simulink model "test(1)"  (R2019a)
settings: Solver=FixedStepAuto  StartTime=0.0  StopTime=inf  RelTol=1e-3
libraries: vexarmcortexlib x23, vexcommonlib x3
settings Model: Creator=hsstudent  LastModifiedBy=hsstudent
settings SolverCC: AutoInsertRateTranBlk=on
settings DataIOCC: LimitDataPoints=on  SignalLoggingSaveFormat=ModelDataLogs  ReturnWorkspaceOutputs=off
settings OptimizationCC: ExpressionDepthLimit=2147483647  LifeSpan=Inf  MaxStackSize=64
settings DebuggingCC: UnderspecifiedInitializationDetection=Classic  MergeDetectMultiDrivingBlocksExec=none  InheritedTsInSrcMsg=none  FcnCallInpInsideContextMsg=warning  UnconnectedInputMsg=none  UnconnectedOutputMsg=none  StateNameClashWarn=warning  SFUnexpectedBacktrackingDiag=warning  SFNoUnconditionalDefaultTransitionDiag=warning  SFExecutionAtInitializationDiag=none  ArithmeticOperatorsInVariantConditions=warning
settings HardwareCC: ProdBitPerPointer=32  ProdBitPerSizeT=32  ProdBitPerPtrDiffT=32  ProdLargestAtomicInteger=Long  ProdLargestAtomicFloat=Double  ProdIntDivRoundTo=Undefined  ProdWordSize=32  ProdHWDeviceType=ARM Compatible->ARM Cortex
settings ModelReferenceCC: PropagateSignalLabelsOutOfModel=off
settings SFSimCC: MATLABDynamicMemAlloc=off
settings RTWCC: SystemTargetFile=ert.tlc  HardwareBoard=ARM Cortex-based VEX Microcontroller  TemplateMakefile=ert_default_tmf  Toolchain=GNU Tools for VEX ARM Cortex
settings CodeAppCC: IgnoreCustomStorageClasses=off  CustomSymbolStrType=$N$R$M  StateflowObjectComments=on  InternalIdentifier=Classic
settings ERTTargetCC: CodeReplacementLibrary=GCC ARM Cortex-M3  MultiwordLength=2048  ConvertIfToSwitch=off  SuppressUnreachableDefaultCases=off

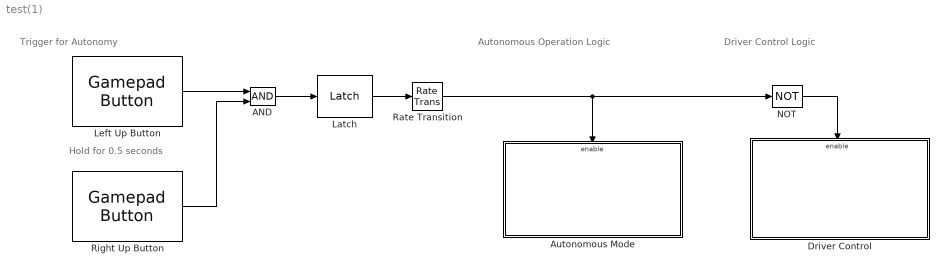
== system test(1) ==
  note: Autonomous Operation Logic
  note: Hold for 0.5 seconds
  note: Driver Control Logic
  note: Trigger for Autonomy
  AND : Logic  IconShape=distinctive  AllPortsSameDT=off  OutDataTypeStr=boolean
  Autonomous Mode : Subsystem
  Driver Control : Subsystem  TreatAsAtomicUnit=on
  Latch : vexcommonlib/Latch  output0=off  BlockPlatform=vexarmcortex
      settings: SourceProductName=Simulink Coder Support Package for ARM Cortex-based VEX Microcontroller  SourceProductBaseCode=EC_VEX_MICRO
  Left Up Button : vexarmcortexlib/Gamepad/Gamepad Button  joystick=1  chan=7  button56=Down  button78=Up  SimulationIn=off  SampleTime=0.5
      settings: SourceProductName=Simulink Coder Support Package for ARM Cortex-based VEX Microcontroller  SourceProductBaseCode=EC_VEX_MICRO
  NOT : Logic  Operator=NOT  IconShape=distinctive  AllPortsSameDT=off  OutDataTypeStr=boolean
  Rate Transition : RateTransition
  Right Up Button : vexarmcortexlib/Gamepad/Gamepad Button  joystick=1  chan=8  button56=Down  button78=Up  SimulationIn=off  SampleTime=0.5
      settings: SourceProductName=Simulink Coder Support Package for ARM Cortex-based VEX Microcontroller  SourceProductBaseCode=EC_VEX_MICRO
  wires:
  AND/1 -> Latch/1
  Rate Transition/1 -> NOT/1, Autonomous Mode/Enable
  Latch/1 -> Rate Transition/1
  Right Up Button/1 -> AND/2
  Left Up Button/1 -> AND/1
  NOT/1 -> Driver Control/Enable

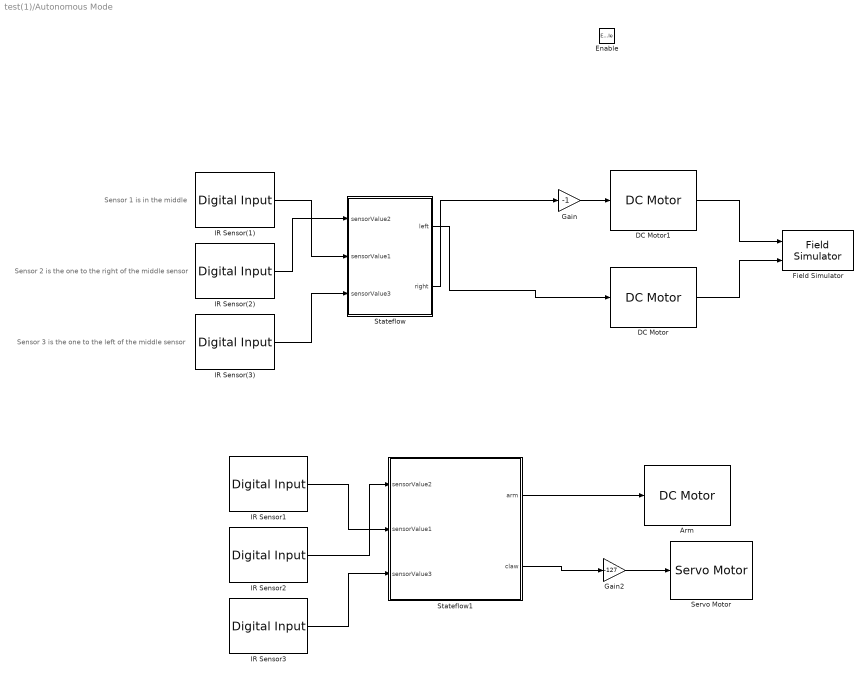
== system test(1)/Autonomous Mode ==
  note: Sensor 3 is the one to the left of the middle sensor
  note: Sensor 2 is the one to the right of the middle sensor
  note: Sensor 1 is in the middle
  Enable : EnablePort  StatesWhenEnabling=reset
  Arm : vexarmcortexlib/Actuators/DC Motor  motor=7  scaleFactor=1/13.5  SimulationOut=on
      settings: SourceProductName=Simulink Coder Support Package for ARM Cortex-based VEX Microcontroller  SourceProductBaseCode=EC_VEX_MICRO
  DC Motor : vexarmcortexlib/Actuators/DC Motor  motor=3  scaleFactor=1/13.5  SimulationOut=on
      settings: SourceProductName=Simulink Coder Support Package for ARM Cortex-based VEX Microcontroller  SourceProductBaseCode=EC_VEX_MICRO
  DC Motor1 : vexarmcortexlib/Actuators/DC Motor  motor=2  scaleFactor=1/13.5  SimulationOut=on
      settings: SourceProductName=Simulink Coder Support Package for ARM Cortex-based VEX Microcontroller  SourceProductBaseCode=EC_VEX_MICRO
  Field Simulator : vexcommonlib/Field Simulator  radius=2.5  space=10  range=200  BlockPlatform=vexarmcortex
      settings: SourceProductName=Simulink Coder Support Package for ARM Cortex-based VEX Microcontroller  SourceProductBaseCode=EC_VEX_MICRO
  Gain : Gain  Gain=-1
  Gain2 : Gain  Gain=-127
  IR Sensor(1) : vexarmcortexlib/Sensors/Digital Input  inChan=9  SimulationIn=off  SampleTime=0.05
      settings: SourceProductName=Simulink Coder Support Package for ARM Cortex-based VEX Microcontroller  SourceProductBaseCode=EC_VEX_MICRO
  IR Sensor(2) : vexarmcortexlib/Sensors/Digital Input  inChan=8  SimulationIn=off  SampleTime=0.05
      settings: SourceProductName=Simulink Coder Support Package for ARM Cortex-based VEX Microcontroller  SourceProductBaseCode=EC_VEX_MICRO
  IR Sensor(3) : vexarmcortexlib/Sensors/Digital Input  inChan=7  SimulationIn=off  SampleTime=0.05
      settings: SourceProductName=Simulink Coder Support Package for ARM Cortex-based VEX Microcontroller  SourceProductBaseCode=EC_VEX_MICRO
  IR Sensor1 : vexarmcortexlib/Sensors/Digital Input  inChan=9  SimulationIn=off  SampleTime=0.05
      settings: SourceProductName=Simulink Coder Support Package for ARM Cortex-based VEX Microcontroller  SourceProductBaseCode=EC_VEX_MICRO
  IR Sensor2 : vexarmcortexlib/Sensors/Digital Input  inChan=8  SimulationIn=off  SampleTime=0.05
      settings: SourceProductName=Simulink Coder Support Package for ARM Cortex-based VEX Microcontroller  SourceProductBaseCode=EC_VEX_MICRO
  IR Sensor3 : vexarmcortexlib/Sensors/Digital Input  inChan=7  SimulationIn=off  SampleTime=0.05
      settings: SourceProductName=Simulink Coder Support Package for ARM Cortex-based VEX Microcontroller  SourceProductBaseCode=EC_VEX_MICRO
  Servo Motor : vexarmcortexlib/Actuators/Servo Motor  motor=4  scaleFactor=60/127  SimulationOut=on
      settings: SourceProductName=Simulink Coder Support Package for ARM Cortex-based VEX Microcontroller  SourceProductBaseCode=EC_VEX_MICRO
  Stateflow : Stateflow chart  TreatAsAtomicUnit=on
  Stateflow1 : Stateflow chart  TreatAsAtomicUnit=on
  wires:
  DC Motor/1 -> Field Simulator/2
  Gain/1 -> DC Motor1/1
  DC Motor1/1 -> Field Simulator/1
  Stateflow/1(left) -> DC Motor/1
  Stateflow/2(right) -> Gain/1
  IR Sensor(1)/1 -> Stateflow/2(sensorValue1)
  IR Sensor1/1 -> Stateflow1/2(sensorValue1)
  IR Sensor2/1 -> Stateflow1/1(sensorValue2)
  IR Sensor3/1 -> Stateflow1/3(sensorValue3)
  Stateflow1/1(arm) -> Arm/1
  Gain2/1 -> Servo Motor/1
  Stateflow1/2(claw) -> Gain2/1
  IR Sensor(2)/1 -> Stateflow/1(sensorValue2)
  IR Sensor(3)/1 -> Stateflow/3(sensorValue3)

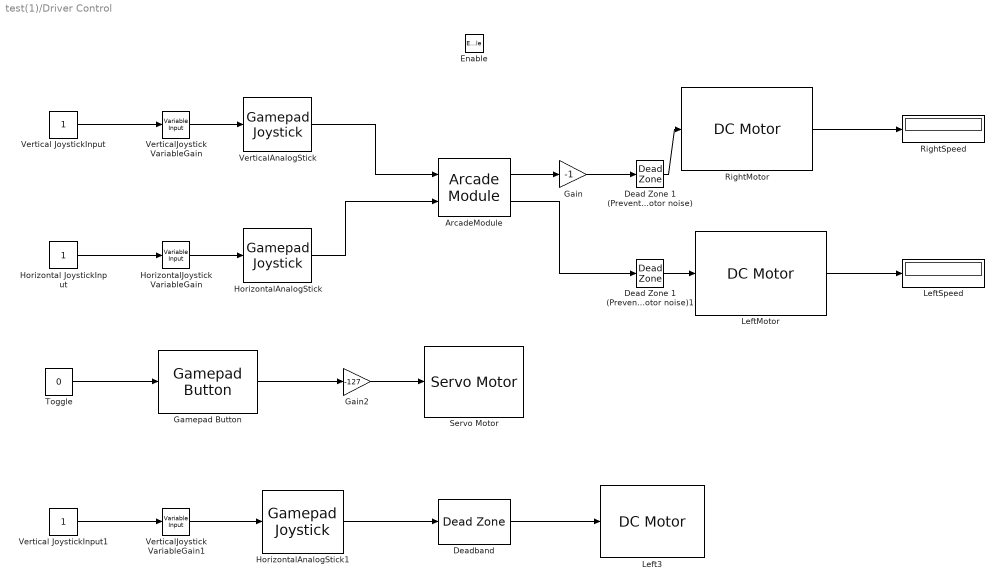
== system test(1)/Driver Control ==
  Enable : EnablePort  StatesWhenEnabling=reset
  ArcadeModule : vexcommonlib/Arcade Module  BlockPlatform=vexarmcortex
      settings: SourceProductName=Simulink Coder Support Package for ARM Cortex-based VEX Microcontroller  SourceProductBaseCode=EC_VEX_MICRO
  Dead Zone 1 (Prevents motor noise) : DeadZone  LowerValue=-30  UpperValue=30  SaturateOnIntegerOverflow=on
  Dead Zone 1 (Prevents motor noise)1 : DeadZone  LowerValue=-30  UpperValue=30  SaturateOnIntegerOverflow=on
  Deadband : DeadZone  SaturateOnIntegerOverflow=on
  Gain : Gain  Gain=-1
  Gain2 : Gain  Gain=-127
  Gamepad Button : vexarmcortexlib/Gamepad/Gamepad Button  joystick=1  chan=7  button56=Up  button78=Down  SimulationIn=on  SampleTime=0.02
      settings: SourceProductName=Simulink Coder Support Package for ARM Cortex-based VEX Microcontroller  SourceProductBaseCode=EC_VEX_MICRO
  Horizontal JoystickInput : Constant
  HorizontalAnalogStick : vexarmcortexlib/Gamepad/Gamepad Joystick  joystick=1  chan=1  SimulationIn=on  SampleTime=0.02
      settings: SourceProductName=Simulink Coder Support Package for ARM Cortex-based VEX Microcontroller  SourceProductBaseCode=EC_VEX_MICRO
  HorizontalAnalogStick1 : vexarmcortexlib/Gamepad/Gamepad Joystick  joystick=1  chan=3  SimulationIn=on  SampleTime=0.02
      settings: SourceProductName=Simulink Coder Support Package for ARM Cortex-based VEX Microcontroller  SourceProductBaseCode=EC_VEX_MICRO
  HorizontalJoystick VariableGain : vexarmcortexlib/Utilities/Variable Input  low=-127  gain=-118.8065  high=127
      settings: SourceProductName=Simulink Coder Support Package for ARM Cortex-based VEX Microcontroller  SourceProductBaseCode=EC_VEX_MICRO
  Left3 : vexarmcortexlib/Actuators/DC Motor  motor=7  scaleFactor=1/13.5  SimulationOut=on
      settings: SourceProductName=Simulink Coder Support Package for ARM Cortex-based VEX Microcontroller  SourceProductBaseCode=EC_VEX_MICRO
  LeftMotor : vexarmcortexlib/Actuators/DC Motor  motor=3  scaleFactor=1/13.5  SimulationOut=on
      settings: SourceProductName=Simulink Coder Support Package for ARM Cortex-based VEX Microcontroller  SourceProductBaseCode=EC_VEX_MICRO
  LeftSpeed : Display
  RightMotor : vexarmcortexlib/Actuators/DC Motor  motor=2  scaleFactor=1/13.5  SimulationOut=on
      settings: SourceProductName=Simulink Coder Support Package for ARM Cortex-based VEX Microcontroller  SourceProductBaseCode=EC_VEX_MICRO
  RightSpeed : Display
  Servo Motor : vexarmcortexlib/Actuators/Servo Motor  motor=4  scaleFactor=60/127  SimulationOut=on
      settings: SourceProductName=Simulink Coder Support Package for ARM Cortex-based VEX Microcontroller  SourceProductBaseCode=EC_VEX_MICRO
  Toggle : Constant  Value=0
      settings: OpenFcn=|
      | if strcmp('0',get_param(gcb, 'Value'))                        set_param(gcb, 'Value', '1');
      | else
      |             set_param(gcb, 'Value', '0');
      | end
  Vertical JoystickInput : Constant
  Vertical JoystickInput1 : Constant
  VerticalAnalogStick : vexarmcortexlib/Gamepad/Gamepad Joystick  joystick=1  chan=2  SimulationIn=on  SampleTime=0.02
      settings: SourceProductName=Simulink Coder Support Package for ARM Cortex-based VEX Microcontroller  SourceProductBaseCode=EC_VEX_MICRO
  VerticalJoystick VariableGain : vexarmcortexlib/Utilities/Variable Input  low=-127  gain=0  high=127
      settings: SourceProductName=Simulink Coder Support Package for ARM Cortex-based VEX Microcontroller  SourceProductBaseCode=EC_VEX_MICRO
  VerticalJoystick VariableGain1 : vexarmcortexlib/Utilities/Variable Input  low=-127  gain=0  high=127
      settings: SourceProductName=Simulink Coder Support Package for ARM Cortex-based VEX Microcontroller  SourceProductBaseCode=EC_VEX_MICRO
  wires:
  Gain2/1 -> Servo Motor/1
  Toggle/1 -> Gamepad Button/1
  Dead Zone 1 (Prevents motor noise)/1 -> RightMotor/1
  VerticalJoystick VariableGain1/1 -> HorizontalAnalogStick1/1
  Vertical JoystickInput1/1 -> VerticalJoystick VariableGain1/1
  Dead Zone 1 (Prevents motor noise)1/1 -> LeftMotor/1
  HorizontalAnalogStick1/1 -> Deadband/1
  ArcadeModule/1 -> Gain/1
  Vertical JoystickInput/1 -> VerticalJoystick VariableGain/1
  VerticalJoystick VariableGain/1 -> VerticalAnalogStick/1
  RightMotor/1 -> RightSpeed/1
  HorizontalJoystick VariableGain/1 -> HorizontalAnalogStick/1
  LeftMotor/1 -> LeftSpeed/1
  ArcadeModule/2 -> Dead Zone 1 (Prevents motor noise)1/1
  Horizontal JoystickInput/1 -> HorizontalJoystick VariableGain/1
  Gamepad Button/1 -> Gain2/1
  Gain/1 -> Dead Zone 1 (Prevents motor noise)/1
  VerticalAnalogStick/1 -> ArcadeModule/1
  HorizontalAnalogStick/1 -> ArcadeModule/2
  Deadband/1 -> Left3/1

== stateflow chart test(1)/Autonomous Mode/Stateflow1 ==
  state Preset
    entry:
    arm = 0;
    claw = 0;
  state TowerDetect
    entry:
    arm = 50;
  state Drop
    entry:
    claw = 1;
    arm = 0;
  state Return
    entry:
    arm = -50;
    claw = 0;
  state Stop
    entry:
    arm = 0;
    claw = 1;
  (default) -> Preset
  TowerDetect -> Drop : after(2,sec)
  Preset -> TowerDetect : [sensorValue1 == 0, sensorValue2 == 0, sensorValue3 == 0]
  Drop -> Return
  Return -> Stop : after(2,sec)
  data: sensorValue2 input; sensorValue1 input; sensorValue3 input; arm output; claw output

== stateflow chart test(1)/Autonomous Mode/Stateflow ==
  state GoForward
    entry:
    left = 100;
    right = 100;
  state Stop
    entry:
    left = 0;
    right= 0;
  state LTurnDetect
    entry:
    right = -100
    left = 100
  state RTurnDetect
    entry:
    right = -100
    left = 100
  state Stop1
    during:
    left = 0
    right = 0
  (default) -> Stop
  Stop -> GoForward : [sensorValue1 == 0]
  GoForward -> LTurnDetect [order 2] : [sensorValue1 == 1, sensorValue2 == 1, sensorValue3 == 0]
  Stop1 -> GoForward : [sensorValue1 == 0]
  GoForward -> RTurnDetect [order 1] : [sensorValue1 == 1, sensorValue2 == 0, sensorValue3 == 1]
  RTurnDetect -> GoForward [order 1] : [sensorValue1 == 0]
  LTurnDetect -> Stop1 : [sensorValue1 == 0]
  RTurnDetect -> Stop1 [order 2] : [sensorValue1 == 0]
  data: left output; right output; sensorValue2 input; sensorValue1 input; sensorValue3 input
